simulink model "sombra_ClP_2"  (R2025a)
settings: Solver=VariableStepAuto  StartTime=0.0  StopTime=inf  RelTol=1e-3
PreLoadFcn:
  | % Caminho dos blocos OPC UA
  | bloco1 = 'sombra_ClP_2/OPC UA Read';
  | bloco2 = 'sombra_ClP_2/OPC UA Read1';
  | 
  | % Verifica configuração do bloco 1
  | policy1 = get_param(bloco1, 'SecurityPolicy');
  | auth1   = get_param(bloco1, 'AuthenticationMode');
  | 
  | if ~strcmp(policy1, 'None') || ~strcmp(auth1, 'Anonymous')
  |     set_param(bloco1, 'SecurityPolicy', 'None', ...
  |                       'AuthenticationMode', 'Anonymous');
  | end
  | 
  | % Verifica configuração do bloco 2
  | policy2 = get_param(bloco2, 'SecurityPolicy');
  | auth2   = get_param(bloco2, 'AuthenticationMode');
  | 
  | if ~strcmp(policy2, 'None') || ~strcmp(auth2, 'Anonymous')
  |     set_param(bloco2, 'SecurityPolicy', 'None', ...
  |                       'AuthenticationMode', 'Anonymous');
  | end
libraries: opcualib x2
settings Model: SimulationMode=accelerator  Creator=guilh  LastModifiedBy=guilh

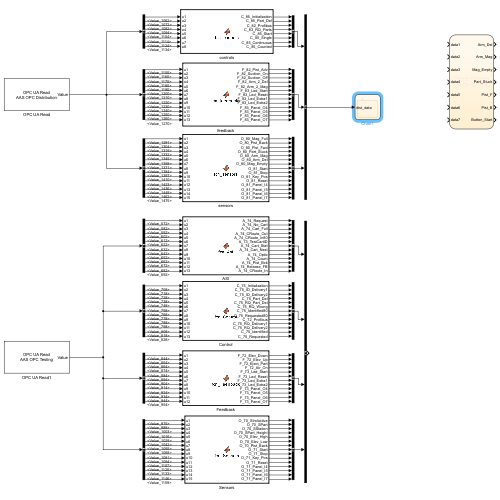
[thumbnail: Simulink's stored preview of the top-level diagram]
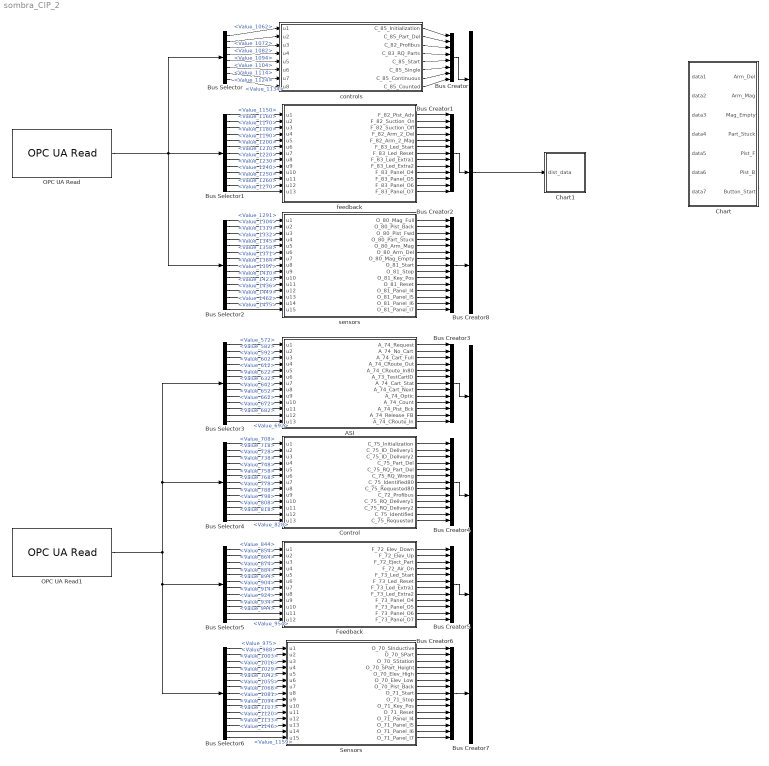
== system sombra_ClP_2 ==
  ASI : MATLAB Function  TreatAsAtomicUnit=on
  Bus Creator : BusCreator  Inputs=8
  Bus Creator1 : BusCreator  Inputs=13
  Bus Creator2 : BusCreator  Inputs=15
  Bus Creator3 : BusCreator  Inputs=13
  Bus Creator4 : BusCreator  Inputs=13
  Bus Creator5 : BusCreator  Inputs=12
  Bus Creator6 : BusCreator  Inputs=15
  Bus Creator7 : BusCreator  Inputs=4
  Bus Creator8 : BusCreator  Inputs=3
  Bus Selector : BusSelector  OutputSignals=Value_1062,Value_1072,Value_1082,Value_1094,Value_1104,Value_1114,Value_1124,Value_1134
  Bus Selector1 : BusSelector  OutputSignals=Value_1150,Value_1160,Value_1170,Value_1180,Value_1190,Value_1200,Value_1210,Value_1220,Value_1230,Value_1240,Value_1250,Value_1260,Value_1270
  Bus Selector2 : BusSelector  OutputSignals=Value_1291,Value_1304,Value_1319,Value_1332,Value_1345,Value_1358,Value_1371,Value_1384,Value_1397,Value_1410,Value_1423,Value_1436,Value_1449,Value_1462,Value_1475
  Bus Selector3 : BusSelector  OutputSignals=Value_572,Value_582,Value_592,Value_602,Value_612,Value_622,Value_632,Value_642,Value_652,Value_662,Value_672,Value_682,Value_692
  Bus Selector4 : BusSelector  OutputSignals=Value_708,Value_718,Value_728,Value_738,Value_748,Value_758,Value_768,Value_778,Value_788,Value_798,Value_808,Value_818,Value_828
  Bus Selector5 : BusSelector  OutputSignals=Value_844,Value_854,Value_864,Value_874,Value_884,Value_894,Value_904,Value_914,Value_924,Value_934,Value_944,Value_954
  Bus Selector6 : BusSelector  OutputSignals=Value_975,Value_988,Value_1003,Value_1016,Value_1029,Value_1042,Value_1055,Value_1068,Value_1081,Value_1094,Value_1107,Value_1120,Value_1133,Value_1146,Value_1159
  Chart : Stateflow chart  TreatAsAtomicUnit=on
  Chart1 : Stateflow chart  TreatAsAtomicUnit=on
  Control : MATLAB Function  TreatAsAtomicUnit=on
  Feedback : MATLAB Function  TreatAsAtomicUnit=on
  OPC UA Read : opcualib/OPC UA Read  SelectedServer=AAS OPC Distribution  ServerList=AAS OPC Distribution  NodeList={ '1', 'Value', '6', '1062', '1'; '2', 'Value', '6', '1072', '1'; '3', 'Value', '6', '1082', '1'; '4', 'Value', '6', '1094', '1'; '5', 'Value', '6', '1104', '1'; '6', 'Value', '6', '1114', '1'; '7', 'Value', '6', '1124', '1'; '8', 'Value', '6', '1134', '1'; '9', 'Value', '6', '1150', '1'; '10', 'Value', '6', '1160', '1'; '11', 'Value', '6', '1170', '1'; '12', 'Value', '6', '1180', '1'; '13', 'Value', '6', '1190', '1'; '14', 'Value', '6', '1200', '1'; '15', 'Value', '6', '1210', '1'; '16', 'Value', '6', '1220', '1'; '17', 'Value', '6', '1230', '1'; '18', 'Value', '6', '1240', '1'; '19', 'Value', '6', '1250', '1'; '20', 'Value', '6', '1260', '1'; '21', 'Value', '6', '1270', '1'; '22', 'Value', '6', '1291', '1'; '23', 'Value', '6', '1304', '1'; '24', 'Value', '6', '1319', '1'; '25', 'Value', '6', '1332', '1'; '26', 'Value', '6', '1345', '1'; '27', 'Value', '6', '1358', '1'; '28', 'Value', '6', '1371', '1'; '29', 'Value', '6', '1384', '1'; '30', 'Value', '6', '1397', '1'; '31', 'Value', '6', '1410', '1'; '32', 'Value', '6', '1423', '1'; '33', 'Value', '6', '1436', '1'; '34', 'Value', '6', '1449', '1'; '35', 'Value', '6', '1462', '1'; '36', 'Value', '6', '1475', '1' }  ShowQualityPort=off  ShowTimestampPort=off  ShowTimestampPortAs=Seconds since start  SampleTime=-1
  OPC UA Read1 : opcualib/OPC UA Read  SelectedServer=AAS OPC Testing  ServerList=AAS OPC Testing  NodeList={ '1', 'Value', '6', '572', '1'; '2', 'Value', '6', '582', '1'; '3', 'Value', '6', '592', '1'; '4', 'Value', '6', '602', '1'; '5', 'Value', '6', '612', '1'; '6', 'Value', '6', '622', '1'; '7', 'Value', '6', '632', '1'; '8', 'Value', '6', '642', '1'; '9', 'Value', '6', '652', '1'; '10', 'Value', '6', '662', '1'; '11', 'Value', '6', '672', '1'; '12', 'Value', '6', '682', '1'; '13', 'Value', '6', '692', '1'; '14', 'Value', '6', '708', '1'; '15', 'Value', '6', '718', '1'; '16', 'Value', '6', '728', '1'; '17', 'Value', '6', '738', '1'; '18', 'Value', '6', '748', '1'; '19', 'Value', '6', '758', '1'; '20', 'Value', '6', '768', '1'; '21', 'Value', '6', '778', '1'; '22', 'Value', '6', '788', '1'; '23', 'Value', '6', '798', '1'; '24', 'Value', '6', '808', '1'; '25', 'Value', '6', '818', '1'; '26', 'Value', '6', '828', '1'; '27', 'Value', '6', '844', '1'; '28', 'Value', '6', '854', '1'; '29', 'Value', '6', '864', '1'; '30', 'Value', '6', '874', '1'; '31', 'Value', '6', '884', '1'; '32', 'Value', '6', '894', '1'; '33', 'Value', '6', '904', '1'; '34', 'Value', '6', '914', '1'; '35', 'Value', '6', '924', '1'; '36', 'Value', '6', '934', '1'; '37', 'Value', '6', '944', '1'; '38', 'Value', '6', '954', '1'; '39', 'Value', '6', '975', '1'; '40', 'Value', '6', '988', '1'; '41', 'Value', '6', '1003', '1'; '42', 'Value', '6', '1016', '1'; '43', 'Value', '6', '1029', '1'; '44', 'Value', '6', '1042', '1'; '45', 'Value', '6', '1055', '1'; '46', 'Value', '6', '1068', '1'; '47', 'Value', '6', '1081', '1'; '48', 'Value', '6', '1094', '1'; '49', 'Value', '6', '1107', '1'; '50', 'Value', '6', '1120', '1'; '51', 'Value', '6', '1133', '1'; '52', 'Value', '6', '1146', '1'; '53', 'Value', '6', '1159', '1' }  ShowQualityPort=off  ShowTimestampPort=off  ShowTimestampPortAs=Seconds since start  SampleTime=-1
  Sensors : MATLAB Function  TreatAsAtomicUnit=on
  controls : MATLAB Function  TreatAsAtomicUnit=on
  feedback : MATLAB Function  TreatAsAtomicUnit=on
  sensors : MATLAB Function  TreatAsAtomicUnit=on
  wires:
  OPC UA Read/1 -> Bus Selector2/1, Bus Selector/1, Bus Selector1/1
  Bus Selector/1 -> controls/1(u1)  "<Value_1062>"
  Bus Selector/2 -> controls/2(u2)  "<Value_1072>"
  Bus Selector/3 -> controls/3(u3)  "<Value_1082>"
  Bus Selector/4 -> controls/4(u4)  "<Value_1094>"
  Bus Selector/5 -> controls/5(u5)  "<Value_1104>"
  Bus Selector/6 -> controls/6(u6)  "<Value_1114>"
  Bus Selector/7 -> controls/7(u7)  "<Value_1124>"
  Bus Selector/8 -> controls/8(u8)  "<Value_1134>"
  Bus Selector1/11 -> feedback/11(u11)  "<Value_1250>"
  Bus Selector1/12 -> feedback/12(u12)  "<Value_1260>"
  Bus Selector1/13 -> feedback/13(u13)  "<Value_1270>"
  Bus Selector1/1 -> feedback/1(u1)  "<Value_1150>"
  Bus Selector1/2 -> feedback/2(u2)  "<Value_1160>"
  Bus Selector1/3 -> feedback/3(u3)  "<Value_1170>"
  Bus Selector1/4 -> feedback/4(u4)  "<Value_1180>"
  Bus Selector1/5 -> feedback/5(u5)  "<Value_1190>"
  Bus Selector1/6 -> feedback/6(u6)  "<Value_1200>"
  Bus Selector1/7 -> feedback/7(u7)  "<Value_1210>"
  Bus Selector1/8 -> feedback/8(u8)  "<Value_1220>"
  Bus Selector1/9 -> feedback/9(u9)  "<Value_1230>"
  Bus Selector1/10 -> feedback/10(u10)  "<Value_1240>"
  Bus Selector2/1 -> sensors/1(u1)  "<Value_1291>"
  Bus Selector2/2 -> sensors/2(u2)  "<Value_1304>"
  Bus Selector2/3 -> sensors/3(u3)  "<Value_1319>"
  Bus Selector2/4 -> sensors/4(u4)  "<Value_1332>"
  Bus Selector2/5 -> sensors/5(u5)  "<Value_1345>"
  Bus Selector2/6 -> sensors/6(u6)  "<Value_1358>"
  Bus Selector2/7 -> sensors/7(u7)  "<Value_1371>"
  Bus Selector2/8 -> sensors/8(u8)  "<Value_1384>"
  Bus Selector2/9 -> sensors/9(u9)  "<Value_1397>"
  Bus Selector2/10 -> sensors/10(u10)  "<Value_1410>"
  Bus Selector2/11 -> sensors/11(u11)  "<Value_1423>"
  Bus Selector2/12 -> sensors/12(u12)  "<Value_1436>"
  Bus Selector2/13 -> sensors/13(u13)  "<Value_1449>"
  Bus Selector2/14 -> sensors/14(u14)  "<Value_1462>"
  Bus Selector2/15 -> sensors/15(u15)  "<Value_1475>"
  OPC UA Read1/1 -> Bus Selector6/1, Bus Selector5/1, Bus Selector3/1, Bus Selector4/1
  Bus Selector3/1 -> ASI/1(u1)  "<Value_572>"
  Bus Selector3/2 -> ASI/2(u2)  "<Value_582>"
  Bus Selector3/3 -> ASI/3(u3)  "<Value_592>"
  Bus Selector3/4 -> ASI/4(u4)  "<Value_602>"
  Bus Selector3/5 -> ASI/5(u5)  "<Value_612>"
  Bus Selector3/6 -> ASI/6(u6)  "<Value_622>"
  Bus Selector3/7 -> ASI/7(u7)  "<Value_632>"
  Bus Selector3/8 -> ASI/8(u8)  "<Value_642>"
  Bus Selector3/9 -> ASI/9(u9)  "<Value_652>"
  Bus Selector3/10 -> ASI/10(u10)  "<Value_662>"
  Bus Selector3/11 -> ASI/11(u11)  "<Value_672>"
  Bus Selector3/12 -> ASI/12(u12)  "<Value_682>"
  Bus Selector3/13 -> ASI/13(u13)  "<Value_692>"
  Bus Selector4/1 -> Control/1(u1)  "<Value_708>"
  Bus Selector4/2 -> Control/2(u2)  "<Value_718>"
  Bus Selector4/3 -> Control/3(u3)  "<Value_728>"
  Bus Selector4/4 -> Control/4(u4)  "<Value_738>"
  Bus Selector4/5 -> Control/5(u5)  "<Value_748>"
  Bus Selector4/6 -> Control/6(u6)  "<Value_758>"
  Bus Selector4/7 -> Control/7(u7)  "<Value_768>"
  Bus Selector4/8 -> Control/8(u8)  "<Value_778>"
  Bus Selector4/9 -> Control/9(u9)  "<Value_788>"
  Bus Selector4/10 -> Control/10(u10)  "<Value_798>"
  Bus Selector4/11 -> Control/11(u11)  "<Value_808>"
  Bus Selector4/12 -> Control/12(u12)  "<Value_818>"
  Bus Selector4/13 -> Control/13(u13)  "<Value_828>"
  Bus Selector5/1 -> Feedback/1(u1)  "<Value_844>"
  Bus Selector5/2 -> Feedback/2(u2)  "<Value_854>"
  Bus Selector5/3 -> Feedback/3(u3)  "<Value_864>"
  Bus Selector5/4 -> Feedback/4(u4)  "<Value_874>"
  Bus Selector5/5 -> Feedback/5(u5)  "<Value_884>"
  Bus Selector5/6 -> Feedback/6(u6)  "<Value_894>"
  Bus Selector5/7 -> Feedback/7(u7)  "<Value_904>"
  Bus Selector5/8 -> Feedback/8(u8)  "<Value_914>"
  Bus Selector5/9 -> Feedback/9(u9)  "<Value_924>"
  Bus Selector5/10 -> Feedback/10(u10)  "<Value_934>"
  Bus Selector5/11 -> Feedback/11(u11)  "<Value_944>"
  Bus Selector5/12 -> Feedback/12(u12)  "<Value_954>"
  Bus Selector6/1 -> Sensors/1(u1)  "<Value_975>"
  Bus Selector6/2 -> Sensors/2(u2)  "<Value_988>"
  Bus Selector6/3 -> Sensors/3(u3)  "<Value_1003>"
  Bus Selector6/4 -> Sensors/4(u4)  "<Value_1016>"
  Bus Selector6/5 -> Sensors/5(u5)  "<Value_1029>"
  Bus Selector6/6 -> Sensors/6(u6)  "<Value_1042>"
  Bus Selector6/7 -> Sensors/7(u7)  "<Value_1055>"
  Bus Selector6/8 -> Sensors/8(u8)  "<Value_1068>"
  Bus Selector6/9 -> Sensors/9(u9)  "<Value_1081>"
  Bus Selector6/10 -> Sensors/10(u10)  "<Value_1094>"
  Bus Selector6/11 -> Sensors/11(u11)  "<Value_1107>"
  Bus Selector6/12 -> Sensors/12(u12)  "<Value_1120>"
  Bus Selector6/13 -> Sensors/13(u13)  "<Value_1133>"
  Bus Selector6/14 -> Sensors/14(u14)  "<Value_1146>"
  Bus Selector6/15 -> Sensors/15(u15)  "<Value_1159>"
  controls/1(C_85_Initialization) -> Bus Creator/1
  controls/2(C_85_Part_Del) -> Bus Creator/2
  controls/3(C_82_Profibus) -> Bus Creator/3
  controls/4(C_83_RQ_Parts) -> Bus Creator/4
  controls/5(C_85_Start) -> Bus Creator/5
  controls/6(C_85_Single) -> Bus Creator/6
  controls/7(C_85_Continuous) -> Bus Creator/7
  controls/8(C_85_Counted) -> Bus Creator/8
  feedback/1(F_82_Pist_Adv) -> Bus Creator1/1
  feedback/2(F_82_Suction_On) -> Bus Creator1/2
  feedback/3(F_82_Suction_Off) -> Bus Creator1/3
  feedback/4(F_82_Arm_2_Del) -> Bus Creator1/4
  feedback/5(F_82_Arm_2_Mag) -> Bus Creator1/5
  feedback/6(F_83_Led_Start) -> Bus Creator1/6
  feedback/7(F_83_Led_Reset) -> Bus Creator1/7
  feedback/8(F_83_Led_Extra1) -> Bus Creator1/8
  feedback/9(F_83_Led_Extra2) -> Bus Creator1/9
  feedback/10(F_83_Panel_O4) -> Bus Creator1/10
  feedback/11(F_83_Panel_O5) -> Bus Creator1/11
  feedback/12(F_83_Panel_O6) -> Bus Creator1/12
  feedback/13(F_83_Panel_O7) -> Bus Creator1/13
  sensors/1(O_80_Mag_Full) -> Bus Creator2/1
  sensors/2(O_80_Pist_Back) -> Bus Creator2/2
  sensors/3(O_80_Pist_Fwd) -> Bus Creator2/3
  sensors/4(O_80_Part_Stuck) -> Bus Creator2/4
  sensors/5(O_80_Arm_Mag) -> Bus Creator2/5
  sensors/6(O_80_Arm_Del) -> Bus Creator2/6
  sensors/7(O_80_Mag_Empty) -> Bus Creator2/7
  sensors/8(O_81_Start) -> Bus Creator2/8
  sensors/9(O_81_Stop) -> Bus Creator2/9
  sensors/10(O_81_Key_Pos) -> Bus Creator2/10
  sensors/11(O_81_Reset) -> Bus Creator2/11
  sensors/12(O_81_Panel_I4) -> Bus Creator2/12
  sensors/13(O_81_Panel_I5) -> Bus Creator2/13
  sensors/14(O_81_Panel_I6) -> Bus Creator2/14
  sensors/15(O_81_Panel_I7) -> Bus Creator2/15
  ASI/1(A_74_Request) -> Bus Creator3/1
  ASI/2(A_74_No_Cart) -> Bus Creator3/2
  ASI/3(A_74_Cart_Full) -> Bus Creator3/3
  ASI/4(A_74_CRoute_Out) -> Bus Creator3/4
  ASI/5(A_74_CRoute_In80) -> Bus Creator3/5
  ASI/6(A_73_TestCartID) -> Bus Creator3/6
  ASI/7(A_74_Cart_Stat) -> Bus Creator3/7
  ASI/8(A_74_Cart_Next) -> Bus Creator3/8
  ASI/9(A_74_Optic) -> Bus Creator3/9
  ASI/10(A_74_Count) -> Bus Creator3/10
  ASI/11(A_74_Pist_Bck) -> Bus Creator3/11
  ASI/12(A_74_Release_FB) -> Bus Creator3/12
  ASI/13(A_74_CRoute_In) -> Bus Creator3/13
  Control/1(C_75_Initialization) -> Bus Creator4/1
  Control/2(C_75_ID_Delivery1) -> Bus Creator4/2
  Control/3(C_75_ID_Delivery2) -> Bus Creator4/3
  Control/4(C_75_Part_Del) -> Bus Creator4/4
  Control/5(C_75_RQ_Part_Del) -> Bus Creator4/5
  Control/6(C_75_RQ_Wrong) -> Bus Creator4/6
  Control/7(C_75_Identified80) -> Bus Creator4/7
  Control/8(C_75_Requested80) -> Bus Creator4/8
  Control/9(C_72_Profibus) -> Bus Creator4/9
  Control/10(C_75_RQ_Delivery1) -> Bus Creator4/10
  Control/11(C_75_RQ_Delivery2) -> Bus Creator4/11
  Control/12(C_75_Identified) -> Bus Creator4/12
  Control/13(C_75_Requested) -> Bus Creator4/13
  Feedback/1(F_72_Elev_Down) -> Bus Creator5/1
  Feedback/2(F_72_Elev_Up) -> Bus Creator5/2
  Feedback/3(F_72_Eject_Part) -> Bus Creator5/3
  Feedback/4(F_72_Air_On) -> Bus Creator5/4
  Feedback/5(F_73_Led_Start) -> Bus Creator5/5
  Feedback/6(F_73_Led_Reset) -> Bus Creator5/6
  Feedback/7(F_73_Led_Extra1) -> Bus Creator5/7
  Feedback/8(F_73_Led_Extra2) -> Bus Creator5/8
  Feedback/9(F_73_Panel_O4) -> Bus Creator5/9
  Feedback/10(F_73_Panel_O5) -> Bus Creator5/10
  Feedback/11(F_73_Panel_O6) -> Bus Creator5/11
  Feedback/12(F_73_Panel_O7) -> Bus Creator5/12
  Sensors/1(O_70_SInductive) -> Bus Creator6/1
  Sensors/2(O_70_SPart) -> Bus Creator6/2
  Sensors/3(O_70_SStation) -> Bus Creator6/3
  Sensors/4(O_70_SPart_Height) -> Bus Creator6/4
  Sensors/5(O_70_Elev_High) -> Bus Creator6/5
  Sensors/6(O_70_Elev_Low) -> Bus Creator6/6
  Sensors/7(O_70_Pist_Back) -> Bus Creator6/7
  Sensors/8(O_71_Start) -> Bus Creator6/8
  Sensors/9(O_71_Stop) -> Bus Creator6/9
  Sensors/10(O_71_Key_Pos) -> Bus Creator6/10
  Sensors/11(O_71_Reset) -> Bus Creator6/11
  Sensors/12(O_71_Panel_I4) -> Bus Creator6/12
  Sensors/13(O_71_Panel_I5) -> Bus Creator6/13
  Sensors/14(O_71_Panel_I6) -> Bus Creator6/14
  Sensors/15(O_71_Panel_I7) -> Bus Creator6/15
  Bus Creator/1 -> Bus Creator8/1
  Bus Creator1/1 -> Bus Creator8/2
  Bus Creator2/1 -> Bus Creator8/3
  Bus Creator6/1 -> Bus Creator7/4
  Bus Creator5/1 -> Bus Creator7/3
  Bus Creator4/1 -> Bus Creator7/2
  Bus Creator3/1 -> Bus Creator7/1
  Bus Creator8/1 -> Chart1/1(dist_data)

== matlab function sombra_ClP_2/sensors ==
  data: u1 input; u2 input; u3 input; u4 input; u5 input; u6 input; u7 input; u8 input; u9 input; u10 input; u11 input; u12 input; u13 input; u14 input; u15 input; O_80_Mag_Full output; O_80_Pist_Back output; O_80_Pist_Fwd output; O_80_Part_Stuck output; O_80_Arm_Mag output; O_80_Arm_Del output; O_80_Mag_Empty output; O_81_Start output; O_81_Stop output; O_81_Key_Pos output; O_81_Reset output; O_81_Panel_I4 output; O_81_Panel_I5 output; O_81_Panel_I6 output; O_81_Panel_I7 output
function [O_80_Mag_Full,O_80_Pist_Back,O_80_Pist_Fwd,O_80_Part_Stuck,...
    O_80_Arm_Mag,O_80_Arm_Del,O_80_Mag_Empty,O_81_Start,O_81_Stop,...
    O_81_Key_Pos,O_81_Reset,O_81_Panel_I4,O_81_Panel_I5,O_81_Panel_I6,...
    O_81_Panel_I7] = fcn_sensors(u1,u2,u3,u4,u5,u6,u7,u8,u9,...
    u10,u11,u12,u13,u14,u15)

O_80_Mag_Full = u1;
O_80_Pist_Back = u2;
O_80_Pist_Fwd = u3;
O_80_Part_Stuck = u4;
O_80_Arm_Mag = u5;
O_80_Arm_Del = u6;
O_80_Mag_Empty = u7;
O_81_Start = u8;
O_81_Stop = u9;
O_81_Key_Pos = u10;
O_81_Reset = u11;
O_81_Panel_I4 = u12;
O_81_Panel_I5 = u13;
O_81_Panel_I6 = u14;
O_81_Panel_I7 = u15;

== matlab function sombra_ClP_2/Control ==
  data: C_75_Initialization output; C_75_ID_Delivery1 output; C_75_ID_Delivery2 output; C_75_Part_Del output; C_75_RQ_Part_Del output; C_75_RQ_Wrong output; C_75_Identified80 output; C_75_Requested80 output; u1 input; C_72_Profibus output; u2 input; u3 input; u4 input; u5 input; u6 input; u7 input; u8 input; u9 input; u10 input; u11 input; u12 input; u13 input; C_75_RQ_Delivery1 output; C_75_RQ_Delivery2 output; C_75_Identified output; C_75_Requested output
function [C_75_Initialization, C_75_ID_Delivery1, C_75_ID_Delivery2, ...
          C_75_Part_Del, C_75_RQ_Part_Del, C_75_RQ_Wrong, C_75_Identified80, ...
          C_75_Requested80, C_72_Profibus, C_75_RQ_Delivery1, C_75_RQ_Delivery2, C_75_Identified, ...
          C_75_Requested] = fcn_Control(u1, u2, u3, u4, u5, u6, u7, u8, u9, u10, u11, u12, u13)

C_75_Initialization = u1;
C_75_ID_Delivery1 = u2;
C_75_ID_Delivery2 = u3;
C_75_Part_Del = u4;
C_75_RQ_Part_Del = u5;
C_75_RQ_Wrong = u6;
C_75_Identified80 = u7;
C_75_Requested80 = u8;
C_72_Profibus = u9;
C_75_RQ_Delivery1 = u10;
C_75_RQ_Delivery2 = u11;
C_75_Identified = u12;
C_75_Requested = u13;

== matlab function sombra_ClP_2/Feedback ==
  data: u1 input; F_72_Elev_Down output; u2 input; u3 input; u4 input; u5 input; u6 input; u7 input; u8 input; u9 input; u10 input; u11 input; u12 input; F_72_Elev_Up output; F_72_Eject_Part output; F_72_Air_On output; F_73_Led_Start output; F_73_Led_Reset output; F_73_Led_Extra1 output; F_73_Led_Extra2 output; F_73_Panel_O4 output; F_73_Panel_O5 output; F_73_Panel_O6 output; F_73_Panel_O7 output
function [F_72_Elev_Down, F_72_Elev_Up, F_72_Eject_Part, F_72_Air_On, ...
          F_73_Led_Start, F_73_Led_Reset, F_73_Led_Extra1, F_73_Led_Extra2, ...
          F_73_Panel_O4, F_73_Panel_O5, F_73_Panel_O6, F_73_Panel_O7] = ...
          fcn_Feedback(u1, u2, u3, u4, u5, u6, u7, u8, u9, u10, u11, u12)

F_72_Elev_Down = u1;
F_72_Elev_Up = u2;
F_72_Eject_Part = u3;
F_72_Air_On = u4;
F_73_Led_Start = u5;
F_73_Led_Reset = u6;
F_73_Led_Extra1 = u7;
F_73_Led_Extra2 = u8;
F_73_Panel_O4 = u9;
F_73_Panel_O5 = u10;
F_73_Panel_O6 = u11;
F_73_Panel_O7 = u12;

== matlab function sombra_ClP_2/Sensors ==
  data: u1 input; O_70_SInductive output; u2 input; u3 input; u4 input; u5 input; u6 input; u7 input; u8 input; u9 input; u10 input; u11 input; u12 input; u13 input; u14 input; u15 input; O_70_SPart output; O_70_SStation output; O_70_SPart_Height output; O_70_Elev_High output; O_70_Elev_Low output; O_70_Pist_Back output; O_71_Start output; O_71_Stop output; O_71_Key_Pos output; O_71_Reset output; O_71_Panel_I4 output; O_71_Panel_I5 output; O_71_Panel_I6 output; O_71_Panel_I7 output
function [O_70_SInductive, O_70_SPart, O_70_SStation, O_70_SPart_Height, ...
          O_70_Elev_High, O_70_Elev_Low, O_70_Pist_Back, O_71_Start, ...
          O_71_Stop, O_71_Key_Pos, O_71_Reset, O_71_Panel_I4, O_71_Panel_I5, ...
          O_71_Panel_I6, O_71_Panel_I7] = ...
          fcn_Sensors(u1, u2, u3, u4, u5, u6, u7, u8, u9, u10, ...
          u11, u12, u13, u14, u15)

O_70_SInductive = u1;
O_70_SPart = u2;
O_70_SStation = u3;
O_70_SPart_Height = u4;
O_70_Elev_High = u5;
O_70_Elev_Low = u6;
O_70_Pist_Back = u7;
O_71_Start = u8;
O_71_Stop = u9;
O_71_Key_Pos = u10;
O_71_Reset = u11;
O_71_Panel_I4 = u12;
O_71_Panel_I5 = u13;
O_71_Panel_I6 = u14;
O_71_Panel_I7 = u15;

== stateflow chart sombra_ClP_2/Chart ==
  state Init
    entry:
    Button_Start = data7;
    Pist_B = data1;
    Pist_F = data2;
    Part_Stuck = data3;
    Arm_Mag = data4;
    Arm_Del = data5;
    Mag_Empty = data6;
  state Arm_2_Del
    entry:
    Pist_B = 1;
    Pist_F = 0;
    Part_Stuck = 0;
    Arm_Mag = 0;
    Arm_Del = 1;
    Mag_Empty = 0;
  state Pist_Fowd
    entry:
    Pist_B = 0;
    Pist_F = 1;
    Part_Stuck = 0;
    Arm_Mag = 0;
    Arm_Del = 1;
    Mag_Empty = 0;
  state Pist_Back
    entry:
    Pist_B = 1;
    Pist_F = 0;
    Part_Stuck = 0;
    Arm_Mag = 0;
    Arm_Del = 1;
    Mag_Empty = 0;
  state Arm_2_Mag
    entry:
    Pist_B = 1;
    Pist_F = 0;
    Part_Stuck = 0;
    Arm_Mag = 1;
    Arm_Del = 0;
    Mag_Empty = 0;
  state Arm_2_Mag1
    entry:
    Button_Start = 0;
    Pist_B = 1;
    Pist_F = 0;
    Part_Stuck = 0;
    Arm_Mag = 1;
    Arm_Del = 0;
    Mag_Empty = 0;
  state Stuck_Off
    entry:
    Pist_B = 1;
    Pist_F = 0;
    Part_Stuck = 0;
    Arm_Mag = 0;
    Arm_Del = 1;
    Mag_Empty = 0;
  state Arm_2_Del1
    entry:
    Pist_B = 1;
    Pist_F = 0;
    Part_Stuck = 1;
    Arm_Mag = 0;
    Arm_Del = 1;
    Mag_Empty = 0;
  state Stuck_On
    entry:
    Pist_B = 1;
    Pist_F = 0;
    Part_Stuck = 1;
    Arm_Mag = 1;
    Arm_Del = 0;
    Mag_Empty = 0;
  (default) -> Init
  Arm_2_Del -> Pist_Fowd : [Arm_Mag == 0 && Arm_Del == 1]
  Pist_Fowd -> Pist_Back : [Pist_B == 0 && Pist_F == 1]
  Pist_Back -> Arm_2_Mag : [Pist_B == 1 && Pist_F == 0]
  Init -> Arm_2_Del : [Button_Start == 1 && Mag_Empty == 0]
  Arm_2_Mag -> Stuck_On : [Arm_Mag == 1 && Arm_Del == 0]
  Arm_2_Del1 -> Stuck_Off : [Arm_Mag == 0 && Arm_Del == 1]
  Stuck_On -> Arm_2_Del1 : [Part_Stuck == 1]
  Stuck_Off -> Arm_2_Mag1 : [Part_Stuck == 0]
  data: data1 input; data2 input; data3 input; data4 input; data5 input; data6 input; Arm_Del output; Arm_Mag output; Mag_Empty output; Part_Stuck output; Pist_F output; Pist_B output; data7 input; Button_Start output

== stateflow chart sombra_ClP_2/Chart1 ==
  state Init
    entry:
    dist_data
    during:
    dist_data
  (default) -> Init
  data: dist_data input

== matlab function sombra_ClP_2/feedback ==
  data: u1 input; F_82_Pist_Adv output; u2 input; u3 input; u4 input; u5 input; u6 input; u7 input; u8 input; u9 input; u10 input; u11 input; u12 input; u13 input; F_82_Suction_On output; F_82_Suction_Off output; F_82_Arm_2_Del output; F_82_Arm_2_Mag output; F_83_Led_Start output; F_83_Led_Reset output; F_83_Led_Extra1 output; F_83_Led_Extra2 output; F_83_Panel_O4 output; F_83_Panel_O5 output; F_83_Panel_O6 output; F_83_Panel_O7 output
function [F_82_Pist_Adv,F_82_Suction_On,F_82_Suction_Off,F_82_Arm_2_Del, ...
    F_82_Arm_2_Mag,F_83_Led_Start,F_83_Led_Reset,F_83_Led_Extra1,...
    F_83_Led_Extra2,F_83_Panel_O4,F_83_Panel_O5,F_83_Panel_O6,...
    F_83_Panel_O7] = fcn_feedbacks(u1,u2,u3,u4,u5,u6,u7,u8,u9,...
    u10,u11,u12,u13)

F_82_Pist_Adv = u1;
F_82_Suction_On = u2;
F_82_Suction_Off = u3;
F_82_Arm_2_Del = u4;
F_82_Arm_2_Mag = u5;
F_83_Led_Start = u6;
F_83_Led_Reset = u7;
F_83_Led_Extra1 = u8;
F_83_Led_Extra2 = u9;
F_83_Panel_O4 = u10;
F_83_Panel_O5 = u11;
F_83_Panel_O6 = u12;
F_83_Panel_O7 = u13;

== matlab function sombra_ClP_2/controls ==
  data: C_85_Initialization output; C_85_Part_Del output; u1 input; u2 input; u3 input; u4 input; u5 input; u6 input; u7 input; C_82_Profibus output; C_83_RQ_Parts output; C_85_Start output; C_85_Single output; C_85_Continuous output; C_85_Counted output; u8 input
function [C_85_Initialization, C_85_Part_Del,...
    C_82_Profibus, C_83_RQ_Parts, ...
    C_85_Start,C_85_Single, C_85_Continuous, ...
    C_85_Counted] = fcn_controls(u1,u2,u3,u4,u5,u6,u7,u8)

C_85_Initialization = u1;
C_85_Part_Del = u2;
C_82_Profibus = u3;
C_83_RQ_Parts = u4;
C_85_Start = u5;
C_85_Single = u6; 
C_85_Continuous = u7;
C_85_Counted = u8;

== matlab function sombra_ClP_2/ASI ==
  data: u1 input; A_74_Request output; u2 input; u3 input; u4 input; u5 input; u6 input; u7 input; u8 input; u9 input; A_74_No_Cart output; A_74_Cart_Full output; A_74_CRoute_Out output; A_74_CRoute_In80 output; A_73_TestCartID output; A_74_Cart_Stat output; A_74_Cart_Next output; A_74_Optic output; A_74_Count output; A_74_Pist_Bck output; A_74_Release_FB output; A_74_CRoute_In output; u10 input; u11 input; u12 input; u13 input
function [A_74_Request, A_74_No_Cart, A_74_Cart_Full, A_74_CRoute_Out,...
    A_74_CRoute_In80, A_73_TestCartID, A_74_Cart_Stat, ...
          A_74_Cart_Next, A_74_Optic, A_74_Count, A_74_Pist_Bck, ...
          A_74_Release_FB,...
          A_74_CRoute_In] = fcn_Asi(u1, u2, u3, u4, u5, u6, u7, u8, u9,...
          u10, u11, u12, u13)

A_74_Request = u1;
A_74_No_Cart = u2;
A_74_Cart_Full = u3;
A_74_CRoute_Out = u4;
A_74_CRoute_In80 = u5;
A_73_TestCartID = u6;
A_74_Cart_Stat = u7;
A_74_Cart_Next = u8;
A_74_Optic = u9;
A_74_Count = u10;
A_74_Pist_Bck = u11;
A_74_Release_FB = u12;
A_74_CRoute_In = u13;
